simulink subsystem "FlowMeter_L_s"  (R2025a)
settings: Solver=VariableStepAuto  StartTime=0.0  StopTime=10.0  RelTol=1e-3
libraries: fl_lib x1, nesl_utility x1
settings Model: Creator=novatehnika  LastModifiedBy=novatehnika

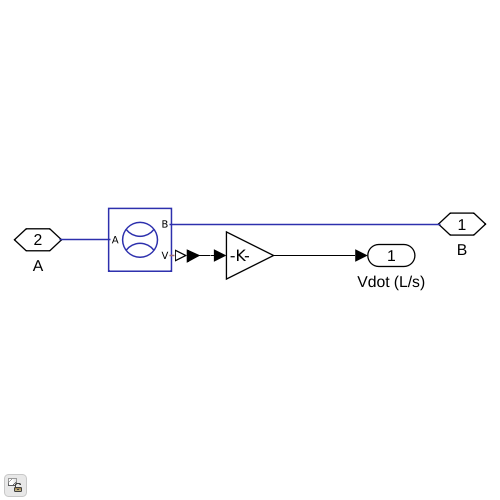
[thumbnail: Simulink's stored preview of the top-level diagram]
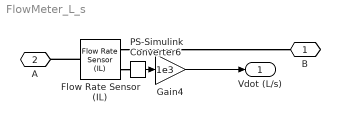
== system FlowMeter_L_s ==
  Flow Rate Sensor (IL) : fl_lib/Isothermal Liquid/Sensors/Flow Rate Sensor (IL)  sensor_type=foundation.enum.mass_volumetric_sensor.volumetric
      settings: InternalSimscapePortConfiguration="{\"Bottom\":[],\"Left\":[{\"id\":\"A\",\"label\":\"A\",\"type\":\"foundation.isothermal_liquid.isothermal_liquid\"}],\"Right\":[{\"id\":\"B\",\"label\":\"B\",\"type\":\"foundation.isothermal_liquid.isothermal_liquid\"},{\"id\":\"V\",\"label\":\"V\",\"type\":\"output\"}],\"Top\":[]}"
  Gain4 : Gain  Gain=1e3
  PS-Simulink Converter6 : nesl_utility/PS-Simulink Converter  PhysicalDomain=network_engine_domain  SubClassName=ps_output  LeftPortType=input  RightPortType=output  PseudoPeriodic=off  Frequencies=[]  VectorFormat=1-D array  Unit=inherit  AffineConversion=off
  B : PMIOPort  Side=Right
  A : PMIOPort  Port=2  Side=Left
  Vdot (L/s) : Outport
  wires:
  PS-Simulink Converter6/1 -> Gain4/1
  Gain4/1 -> Vdot (L/s)/1
  connections:
  Flow Rate Sensor (IL)/RConn2 -- PS-Simulink Converter6/LConn1
  Flow Rate Sensor (IL)/RConn1 -- B/RConn1
  Flow Rate Sensor (IL)/LConn1 -- A/RConn1
